simulink library "HybridSimLib"  (Simulink 7.9)
settings: Solver=ode45  SolverMode=SingleTasking  StartTime=0.0  StopTime=10.0  RelTol=1e-3
undefined symbols (not defined in the file or in its folder): DiscIntNeverNeededParam, HybridCtrlParameters, newTarget, targDsp
libraries: simulink x10, xpclib x7
settings Model: Creator=Andreas Schellenberg  LastModifiedBy=Andreas

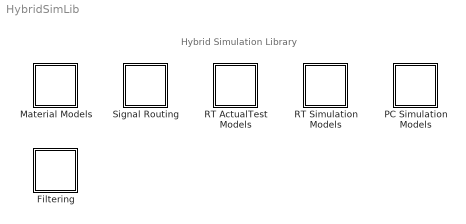
== system HybridSimLib ==
  note: Hybrid Simulation Library
  Filtering : Subsystem
  Material Models : Subsystem
  PC Simulation Models : Subsystem
  RT ActualTest Models : Subsystem
  RT Simulation Models : Subsystem
  Signal Routing : Subsystem

== system HybridSimLib/Filtering ==
  note: Filtering Blocks
  MovingAverage Filter : DiscreteFir  Coefficients=1/numSample*ones(1,numSample)  mask(Moving Average Filter){numSample=5}
      mask prompts: numSample "Number of Samples: numSample"
      mask help:
      | Moving average filter by using discrete FIR filter.
      | Set numSample = 1 for no filtering.
      mask Display: fprintf('MovingAverage\nFilter')
  median filter : S-Function  FunctionName=medianFilter  Parameters=width  EnableBusSupport=off  mask(Moving Median Filter){width=1}
      mask prompts: width "Glitch width (samples)"
      mask Display: fprintf('MovingMedian\nFilter')

== system HybridSimLib/Material Models ==
  note: Material Model Blocks
  continuousD : Subsystem  mask(Continuous Bouc-Wen Model){k=, fy=, alpha=, beta=0.5, gamma=0.5, n=1.0}
      mask prompts: k "Elastic Stiffness: k"; fy "Yield Strength: fy"; alpha "Post-Yield Stiffness Ratio: alpha"; beta "Hysteresis Shape Parameter: beta"; gamma "Hysteresis Shape Parameter: gamma"; n "Smoothness of Transition Parameter: n"
      mask help: Continuous model using displacement inputs to produce force outputs.
      mask Display: disp('Bouc-Wen\nModel')
  continuousDV : Subsystem  mask(Continuous Bouc-Wen Model){k=, fy=, alpha=, beta=0.5, gamma=0.5, n=1.0}
      mask prompts: k "Elastic Stiffness: k"; fy "Yield Strength: fy"; alpha "Post-Yield Stiffness Ratio: alpha"; beta "Hysteresis Shape Parameter: beta"; gamma "Hysteresis Shape Parameter: gamma"; n "Smoothness of Transition Parameter: n"
      mask help: Continuous model using displacement and velocity inputs to produce force outputs.
      mask Display: disp('Bouc-Wen\nModel')
  discreteD : Subsystem  mask(Discrete Bouc-Wen Model){k=, fy=, alpha=, beta=, gamma=0.5, n=0.5, dt=1.0}
      mask prompts: k "Elastic Stiffness: k"; fy "Yield Strength: fy"; alpha "Post-Yield Stiffness Ratio: alpha"; beta "Hysteresis Shape Parameter: beta"; gamma "Hysteresis Shape Parameter: gamma"; n "Smoothness of Transition Parameter: n"; dt "Sample time: dt"
      mask help: Discrete model using displacement inputs to produce force outputs.
      mask Display: disp('Bouc-Wen\nModel')
  discreteDV : Subsystem  mask(Discrete Bouc-Wen Model){k=, fy=, alpha=, beta=0.5, gamma=0.5, n=1.0}
      mask prompts: k "Elastic Stiffness: k"; fy "Yield Strength: fy"; alpha "Post-Yield Stiffness Ratio: alpha"; beta "Hysteresis Shape Parameter: beta"; gamma "Hysteresis Shape Parameter: gamma"; n "Smoothness of Transition Parameter: n"
      mask help: Discrete model using displacement and velocity inputs to produce force outputs.
      mask Display: disp('Bouc-Wen\nModel')

== system HybridSimLib/PC Simulation Models ==
  note: PC Simulation Models
  cmAPI dSpace : Subsystem
  cmAPI xPCTarget STS : Subsystem

== system HybridSimLib/RT ActualTest Models ==
  note: Real Time ActualTest Models
  cmAPI dSpace : Subsystem
  cmAPI xPCTarget STS : Subsystem

== system HybridSimLib/RT Simulation Models ==
  note: Real Time Simulation Models
  cmAPI dSpace : Subsystem
  cmAPI xPCTarget STS : Subsystem

== system HybridSimLib/Signal Routing ==
  note: Signal Routing Blocks
  Offset : Subsystem  mask(Signal Offset){nS=[], nOffset=[], dt=[]}
      mask prompts: nS "Number of Signals: nS"; nOffset "Number of samples to initialize offset: nOffset"; dt "Sample time: dt"
      mask help:
      | Offset signal by average of signal over initial number of samples.
      | Set nOffset = -1 for no signal offset.
      mask Display: fprintf('Signal\nOffset')
  assemble : Subsystem  mask(to Actuators){id=, size=}
      mask prompts: id "Index Vector: id"; size "Vector Size: size"
      mask help: To select to which actuator(s) the signals are going to
      mask Display: disp('Assemble')
  extract : Subsystem  mask(from Actuators){id=, size=}
      mask prompts: id "Index Vector: id"; size "Vector Size: size"
      mask help: To select from which actuator(s) the signals are coming from
      mask Display: disp('Extract')

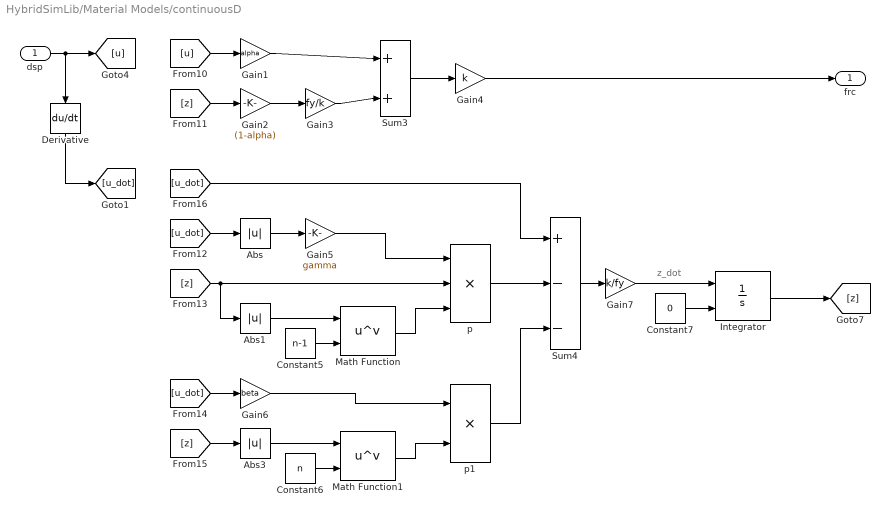
== system HybridSimLib/Material Models/continuousD ==
  note: z_dot
  dsp : Inport
  Abs : Abs  SaturateOnIntegerOverflow=on
  Abs1 : Abs  SaturateOnIntegerOverflow=on
  Abs3 : Abs  SaturateOnIntegerOverflow=on
  Constant5 : Constant  Value=n-1
  Constant6 : Constant  Value=n
  Constant7 : Constant  Value=0
  Derivative : Derivative
  Gain1 : Gain  Gain=alpha  SaturateOnIntegerOverflow=on  OutDataTypeStr=Inherit: Same as input  ParamDataTypeStr=Inherit: Same as input
  Gain2 : Gain  Gain=(1-alpha)  SaturateOnIntegerOverflow=on  OutDataTypeStr=Inherit: Same as input  ParamDataTypeStr=Inherit: Same as input
  Gain3 : Gain  Gain=fy/k  SaturateOnIntegerOverflow=on  OutDataTypeStr=Inherit: Same as input  ParamDataTypeStr=Inherit: Same as input
  Gain4 : Gain  Gain=k  SaturateOnIntegerOverflow=on  OutDataTypeStr=Inherit: Same as input  ParamDataTypeStr=Inherit: Same as input
  Gain5 : Gain  Gain=gamma  SaturateOnIntegerOverflow=on  OutDataTypeStr=Inherit: Same as input  ParamDataTypeStr=Inherit: Same as input
  Gain6 : Gain  Gain=beta  SaturateOnIntegerOverflow=on  OutDataTypeStr=Inherit: Same as input  ParamDataTypeStr=Inherit: Same as input
  Gain7 : Gain  Gain=k/fy  SaturateOnIntegerOverflow=on  OutDataTypeStr=Inherit: Same as input  ParamDataTypeStr=Inherit: Same as input
  Integrator : Integrator  InitialConditionSource=external
  Math Function : Math  Operator=pow  SaturateOnIntegerOverflow=on
  Math Function1 : Math  Operator=pow  SaturateOnIntegerOverflow=on
  Sum3 : Sum  Inputs=+|+  SaturateOnIntegerOverflow=on  InputSameDT=on  OutDataTypeStr=Inherit: Same as first input
  Sum4 : Sum  Inputs=+|-|-  SaturateOnIntegerOverflow=on  InputSameDT=on  OutDataTypeStr=Inherit: Same as first input
  p : Product  Inputs=***  SaturateOnIntegerOverflow=on  InputSameDT=on  OutDataTypeStr=Inherit: Same as first input
  p1 : Product  Inputs=**  SaturateOnIntegerOverflow=on  InputSameDT=on  OutDataTypeStr=Inherit: Same as first input
  frc : Outport
  wires:
  [u] -> Gain1/1
  Gain2/1 -> Gain3/1
  [z] -> Gain2/1
  Gain3/1 -> Sum3/2
  Gain1/1 -> Sum3/1
  Sum3/1 -> Gain4/1
  Gain4/1 -> frc/1
  [u_dot] -> Abs/1
  [z] -> p/2, Abs1/1
  Abs/1 -> Gain5/1
  Abs1/1 -> Math Function/1
  Constant5/1 -> Math Function/2
  Gain5/1 -> p/1
  Math Function/1 -> p/3
  [z] -> Abs3/1
  [u_dot] -> Gain6/1
  Abs3/1 -> Math Function1/1
  Constant6/1 -> Math Function1/2
  Gain6/1 -> p1/1
  Math Function1/1 -> p1/2
  p/1 -> Sum4/2
  p1/1 -> Sum4/3
  [u_dot] -> Sum4/1
  Constant7/1 -> Integrator/2
  Sum4/1 -> Gain7/1
  Integrator/1 -> [z]
  dsp/1 -> [u], Derivative/1
  Derivative/1 -> [u_dot]
  Gain7/1 -> Integrator/1

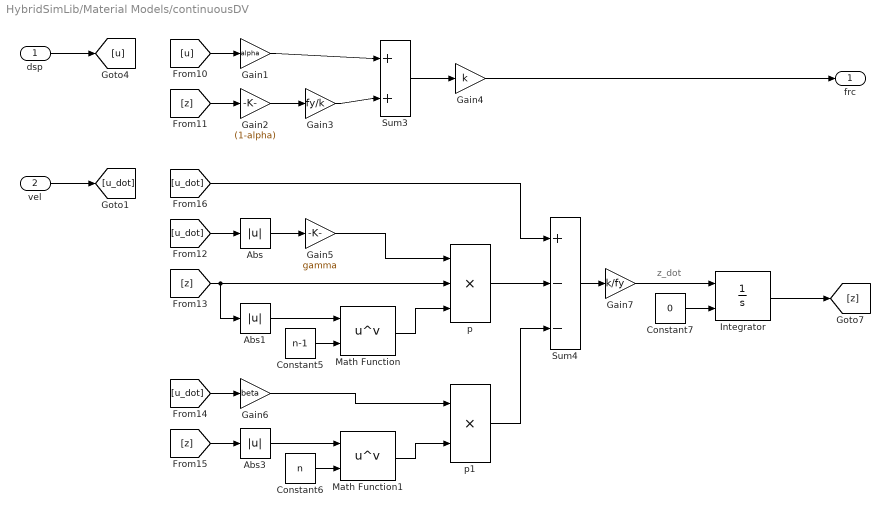
== system HybridSimLib/Material Models/continuousDV ==
  note: z_dot
  dsp : Inport
  vel : Inport  Port=2
  Abs : Abs  SaturateOnIntegerOverflow=on
  Abs1 : Abs  SaturateOnIntegerOverflow=on
  Abs3 : Abs  SaturateOnIntegerOverflow=on
  Constant5 : Constant  Value=n-1
  Constant6 : Constant  Value=n
  Constant7 : Constant  Value=0
  Gain1 : Gain  Gain=alpha  SaturateOnIntegerOverflow=on  OutDataTypeStr=Inherit: Same as input  ParamDataTypeStr=Inherit: Same as input
  Gain2 : Gain  Gain=(1-alpha)  SaturateOnIntegerOverflow=on  OutDataTypeStr=Inherit: Same as input  ParamDataTypeStr=Inherit: Same as input
  Gain3 : Gain  Gain=fy/k  SaturateOnIntegerOverflow=on  OutDataTypeStr=Inherit: Same as input  ParamDataTypeStr=Inherit: Same as input
  Gain4 : Gain  Gain=k  SaturateOnIntegerOverflow=on  OutDataTypeStr=Inherit: Same as input  ParamDataTypeStr=Inherit: Same as input
  Gain5 : Gain  Gain=gamma  SaturateOnIntegerOverflow=on  OutDataTypeStr=Inherit: Same as input  ParamDataTypeStr=Inherit: Same as input
  Gain6 : Gain  Gain=beta  SaturateOnIntegerOverflow=on  OutDataTypeStr=Inherit: Same as input  ParamDataTypeStr=Inherit: Same as input
  Gain7 : Gain  Gain=k/fy  SaturateOnIntegerOverflow=on  OutDataTypeStr=Inherit: Same as input  ParamDataTypeStr=Inherit: Same as input
  Integrator : Integrator  InitialConditionSource=external
  Math Function : Math  Operator=pow  SaturateOnIntegerOverflow=on
  Math Function1 : Math  Operator=pow  SaturateOnIntegerOverflow=on
  Sum3 : Sum  Inputs=+|+  SaturateOnIntegerOverflow=on  InputSameDT=on  OutDataTypeStr=Inherit: Same as first input
  Sum4 : Sum  Inputs=+|-|-  SaturateOnIntegerOverflow=on  InputSameDT=on  OutDataTypeStr=Inherit: Same as first input
  p : Product  Inputs=***  SaturateOnIntegerOverflow=on  InputSameDT=on  OutDataTypeStr=Inherit: Same as first input
  p1 : Product  Inputs=**  SaturateOnIntegerOverflow=on  InputSameDT=on  OutDataTypeStr=Inherit: Same as first input
  frc : Outport
  wires:
  Gain7/1 -> Integrator/1
  dsp/1 -> [u]
  Integrator/1 -> [z]
  Sum4/1 -> Gain7/1
  Constant7/1 -> Integrator/2
  [u_dot] -> Sum4/1
  p1/1 -> Sum4/3
  p/1 -> Sum4/2
  Math Function1/1 -> p1/2
  Gain6/1 -> p1/1
  Constant6/1 -> Math Function1/2
  Abs3/1 -> Math Function1/1
  [u_dot] -> Gain6/1
  [z] -> Abs3/1
  Math Function/1 -> p/3
  Gain5/1 -> p/1
  Constant5/1 -> Math Function/2
  Abs1/1 -> Math Function/1
  Abs/1 -> Gain5/1
  [z] -> Abs1/1, p/2
  [u_dot] -> Abs/1
  Gain4/1 -> frc/1
  Sum3/1 -> Gain4/1
  Gain1/1 -> Sum3/1
  Gain3/1 -> Sum3/2
  [z] -> Gain2/1
  Gain2/1 -> Gain3/1
  [u] -> Gain1/1
  vel/1 -> [u_dot]

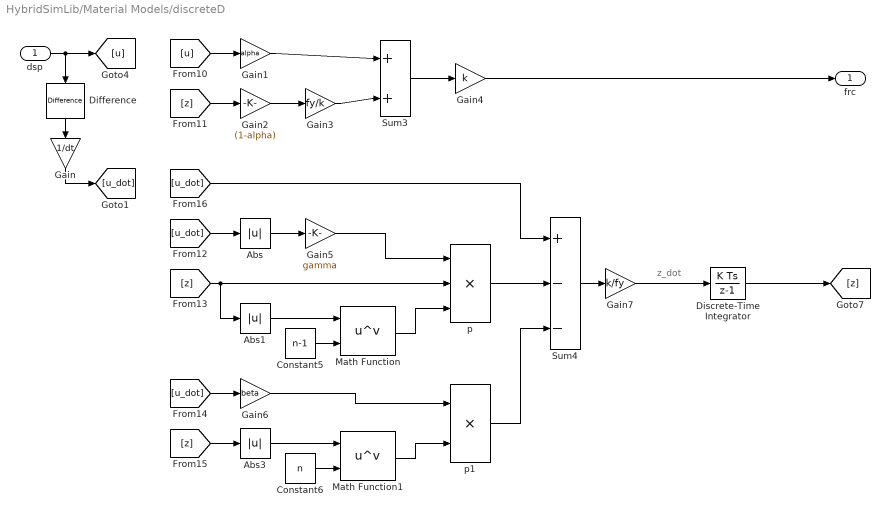
== system HybridSimLib/Material Models/discreteD ==
  note: z_dot
  dsp : Inport
  Abs : Abs  SaturateOnIntegerOverflow=on
  Abs1 : Abs  SaturateOnIntegerOverflow=on
  Abs3 : Abs  SaturateOnIntegerOverflow=on
  Constant5 : Constant  Value=n-1
  Constant6 : Constant  Value=n
  Difference : simulink/Discrete/Difference  ICPrevInput=0.0  InputProcessing=Inherited  OutMin=[]  OutMax=[]  OutDataType=sfix(16)  OutScaling=2^-10  DoSatur=off
  Discrete-Time Integrator : DiscreteIntegrator  SampleTime=-1  ICPrevOutput=DiscIntNeverNeededParam  ICPrevScaledInput=DiscIntNeverNeededParam
  Gain : Gain  Gain=1/dt
  Gain1 : Gain  Gain=alpha  SaturateOnIntegerOverflow=on  OutDataTypeStr=Inherit: Same as input  ParamDataTypeStr=Inherit: Same as input
  Gain2 : Gain  Gain=(1-alpha)  SaturateOnIntegerOverflow=on  OutDataTypeStr=Inherit: Same as input  ParamDataTypeStr=Inherit: Same as input
  Gain3 : Gain  Gain=fy/k  SaturateOnIntegerOverflow=on  OutDataTypeStr=Inherit: Same as input  ParamDataTypeStr=Inherit: Same as input
  Gain4 : Gain  Gain=k  SaturateOnIntegerOverflow=on  OutDataTypeStr=Inherit: Same as input  ParamDataTypeStr=Inherit: Same as input
  Gain5 : Gain  Gain=gamma  SaturateOnIntegerOverflow=on  OutDataTypeStr=Inherit: Same as input  ParamDataTypeStr=Inherit: Same as input
  Gain6 : Gain  Gain=beta  SaturateOnIntegerOverflow=on  OutDataTypeStr=Inherit: Same as input  ParamDataTypeStr=Inherit: Same as input
  Gain7 : Gain  Gain=k/fy  SaturateOnIntegerOverflow=on  OutDataTypeStr=Inherit: Same as input  ParamDataTypeStr=Inherit: Same as input
  Math Function : Math  Operator=pow  SaturateOnIntegerOverflow=on
  Math Function1 : Math  Operator=pow  SaturateOnIntegerOverflow=on
  Sum3 : Sum  Inputs=+|+  SaturateOnIntegerOverflow=on  InputSameDT=on  OutDataTypeStr=Inherit: Same as first input
  Sum4 : Sum  Inputs=+|-|-  SaturateOnIntegerOverflow=on  InputSameDT=on  OutDataTypeStr=Inherit: Same as first input
  p : Product  Inputs=***  SaturateOnIntegerOverflow=on  InputSameDT=on  OutDataTypeStr=Inherit: Same as first input
  p1 : Product  Inputs=**  SaturateOnIntegerOverflow=on  InputSameDT=on  OutDataTypeStr=Inherit: Same as first input
  frc : Outport
  wires:
  [u] -> Gain1/1
  Gain2/1 -> Gain3/1
  [z] -> Gain2/1
  Gain3/1 -> Sum3/2
  Gain1/1 -> Sum3/1
  Sum3/1 -> Gain4/1
  Gain4/1 -> frc/1
  [u_dot] -> Abs/1
  [z] -> p/2, Abs1/1
  Abs/1 -> Gain5/1
  Abs1/1 -> Math Function/1
  Constant5/1 -> Math Function/2
  Gain5/1 -> p/1
  Math Function/1 -> p/3
  [z] -> Abs3/1
  [u_dot] -> Gain6/1
  Abs3/1 -> Math Function1/1
  Constant6/1 -> Math Function1/2
  Gain6/1 -> p1/1
  Math Function1/1 -> p1/2
  p/1 -> Sum4/2
  p1/1 -> Sum4/3
  [u_dot] -> Sum4/1
  Sum4/1 -> Gain7/1
  Discrete-Time Integrator/1 -> [z]
  dsp/1 -> [u], Difference/1
  Gain7/1 -> Discrete-Time Integrator/1
  Difference/1 -> Gain/1
  Gain/1 -> [u_dot]

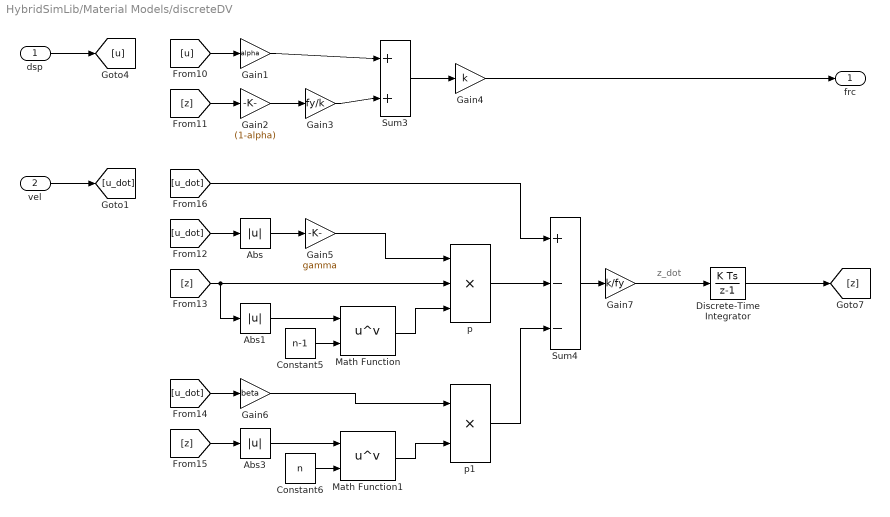
== system HybridSimLib/Material Models/discreteDV ==
  note: z_dot
  dsp : Inport
  vel : Inport  Port=2
  Abs : Abs  SaturateOnIntegerOverflow=on
  Abs1 : Abs  SaturateOnIntegerOverflow=on
  Abs3 : Abs  SaturateOnIntegerOverflow=on
  Constant5 : Constant  Value=n-1
  Constant6 : Constant  Value=n
  Discrete-Time Integrator : DiscreteIntegrator  SampleTime=-1  ICPrevOutput=DiscIntNeverNeededParam  ICPrevScaledInput=DiscIntNeverNeededParam
  Gain1 : Gain  Gain=alpha  SaturateOnIntegerOverflow=on  OutDataTypeStr=Inherit: Same as input  ParamDataTypeStr=Inherit: Same as input
  Gain2 : Gain  Gain=(1-alpha)  SaturateOnIntegerOverflow=on  OutDataTypeStr=Inherit: Same as input  ParamDataTypeStr=Inherit: Same as input
  Gain3 : Gain  Gain=fy/k  SaturateOnIntegerOverflow=on  OutDataTypeStr=Inherit: Same as input  ParamDataTypeStr=Inherit: Same as input
  Gain4 : Gain  Gain=k  SaturateOnIntegerOverflow=on  OutDataTypeStr=Inherit: Same as input  ParamDataTypeStr=Inherit: Same as input
  Gain5 : Gain  Gain=gamma  SaturateOnIntegerOverflow=on  OutDataTypeStr=Inherit: Same as input  ParamDataTypeStr=Inherit: Same as input
  Gain6 : Gain  Gain=beta  SaturateOnIntegerOverflow=on  OutDataTypeStr=Inherit: Same as input  ParamDataTypeStr=Inherit: Same as input
  Gain7 : Gain  Gain=k/fy  SaturateOnIntegerOverflow=on  OutDataTypeStr=Inherit: Same as input  ParamDataTypeStr=Inherit: Same as input
  Math Function : Math  Operator=pow  SaturateOnIntegerOverflow=on
  Math Function1 : Math  Operator=pow  SaturateOnIntegerOverflow=on
  Sum3 : Sum  Inputs=+|+  SaturateOnIntegerOverflow=on  InputSameDT=on  OutDataTypeStr=Inherit: Same as first input
  Sum4 : Sum  Inputs=+|-|-  SaturateOnIntegerOverflow=on  InputSameDT=on  OutDataTypeStr=Inherit: Same as first input
  p : Product  Inputs=***  SaturateOnIntegerOverflow=on  InputSameDT=on  OutDataTypeStr=Inherit: Same as first input
  p1 : Product  Inputs=**  SaturateOnIntegerOverflow=on  InputSameDT=on  OutDataTypeStr=Inherit: Same as first input
  frc : Outport
  wires:
  vel/1 -> [u_dot]
  [u] -> Gain1/1
  Gain2/1 -> Gain3/1
  [z] -> Gain2/1
  Gain3/1 -> Sum3/2
  Gain1/1 -> Sum3/1
  Sum3/1 -> Gain4/1
  Gain4/1 -> frc/1
  [u_dot] -> Abs/1
  [z] -> p/2, Abs1/1
  Abs/1 -> Gain5/1
  Abs1/1 -> Math Function/1
  Constant5/1 -> Math Function/2
  Gain5/1 -> p/1
  Math Function/1 -> p/3
  [z] -> Abs3/1
  [u_dot] -> Gain6/1
  Abs3/1 -> Math Function1/1
  Constant6/1 -> Math Function1/2
  Gain6/1 -> p1/1
  Math Function1/1 -> p1/2
  p/1 -> Sum4/2
  p1/1 -> Sum4/3
  [u_dot] -> Sum4/1
  Sum4/1 -> Gain7/1
  Discrete-Time Integrator/1 -> [z]
  dsp/1 -> [u]
  Gain7/1 -> Discrete-Time Integrator/1

== system HybridSimLib/PC Simulation Models/cmAPI dSpace ==
  note: cmAPI-dSpace Blocks

== system HybridSimLib/PC Simulation Models/cmAPI xPCTarget STS ==
  note: cmAPI-xPCTarget-STS Blocks

== system HybridSimLib/RT ActualTest Models/cmAPI dSpace ==
  note: cmAPI-dSpace Blocks
  dSpace HC : Subsystem  mask(Hybrid Controller: D3/D3){nAct=1, dtInt=HybridCtrlParameters.dtInt, dtSim=HybridCtrlParameters.dtSim, dtCon=HybridCtrlParameters.dtCon, N=HybridCtrlParameters.N, iDelay=HybridCtrlParameters.iDelay, dspLim=HybridCtrlParameters.dspLim, velLim=HybridCtrlParameters.velLim}
      mask prompts: nAct "Number of Actuators: nAct"; dtInt "Integration time step: dtInt"; dtSim "Simulation time step: dtSim"; dtCon "Controller time step: dtCon"; N "Maximum number of substeps: N"; iDelay "Number of delay steps: iDelay"; dspLim "Displacement limit: dspLim"; velLim "Velocity limit: velLim"
      mask help: Hybrid Controller using C0-continuous cubic Lagrange interpolation for prediction and correction
      mask Display: disp('dSpace\nHybrid Controller\n(D3/D3)')

== system HybridSimLib/RT ActualTest Models/cmAPI xPCTarget STS ==
  note: cmAPI-xPCTarget-STS Blocks
  xPC HC : Subsystem  mask(Hybrid Controller: D3/D3){nAct=1, dtInt=HybridCtrlParameters.dtInt, dtSim=HybridCtrlParameters.dtSim, dtCon=HybridCtrlParameters.dtCon, N=HybridCtrlParameters.N, iDelay=HybridCtrlParameters.iDelay}
      mask prompts: nAct "Number of Actuators: nAct"; dtInt "Integration time step: dtInt"; dtSim "Simulation time step: dtSim"; dtCon "Controller time step: dtCon"; N "Maximum number of substeps: N"; iDelay "Number of delay steps: iDelay"
      mask help: Hybrid Controller using C0-continuous cubic Lagrange interpolation for prediction and correction
      mask Display: disp('xPC Target\nHybrid Controller\n(D3/D3)')

== system HybridSimLib/RT Simulation Models/cmAPI dSpace ==
  note: cmAPI-dSpace Blocks

== system HybridSimLib/RT Simulation Models/cmAPI xPCTarget STS ==
  note: cmAPI-xPCTarget-STS Blocks

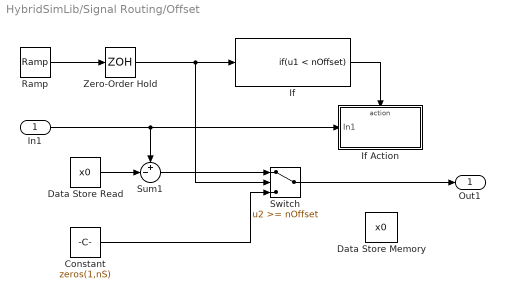
== system HybridSimLib/Signal Routing/Offset ==
  In1 : Inport
  Constant : Constant  Value=zeros(1,nS)
  Data Store Memory : DataStoreMemory  DataStoreName=x0  InitialValue=zeros(1,nS)  OutDataTypeStr=double
  Data Store Read : DataStoreRead  DataStoreName=x0  SampleTime=dt
  If : If  IfExpression=u1 < nOffset  ShowElse=off
  If Action : Subsystem  TreatAsAtomicUnit=on
  Ramp : simulink/Sources/Ramp  slope=1/dt  start=0  X0=0
  Sum1 : Sum  Inputs=+-|  SaturateOnIntegerOverflow=on  InputSameDT=on  OutDataTypeStr=Inherit: Same as first input
  Switch : Switch  Threshold=nOffset  SaturateOnIntegerOverflow=on  InputSameDT=on
  Zero-Order Hold : ZeroOrderHold  SampleTime=dt
  Out1 : Outport
  wires:
  Ramp/1 -> Zero-Order Hold/1
  If/1 -> If Action/Action
  Zero-Order Hold/1 -> If/1, Switch/2
  Constant/1 -> Switch/3
  In1/1 -> Sum1/1, If Action/1(In1)
  Data Store Read/1 -> Sum1/2
  Sum1/1 -> Switch/1
  Switch/1 -> Out1/1

== system HybridSimLib/Signal Routing/assemble ==
  In1 : Inport
  Assignment : Assignment  OutputInitialize=Specify size for each dimension in table  IndexOptions=Index vector (port)  Indices=1  OutputSizes=size
  Constant : Constant  Value=id
  Out1 : Outport
  wires:
  In1/1 -> Assignment/1
  Assignment/1 -> Out1/1
  Constant/1 -> Assignment/2

== system HybridSimLib/Signal Routing/extract ==
  In1 : Inport
  Selector : Selector  InputPortWidth=size  IndexOptions=Index vector (dialog)  Indices=id  OutputSizes=1
  Out1 : Outport
  wires:
  In1/1 -> Selector/1
  Selector/1 -> Out1/1

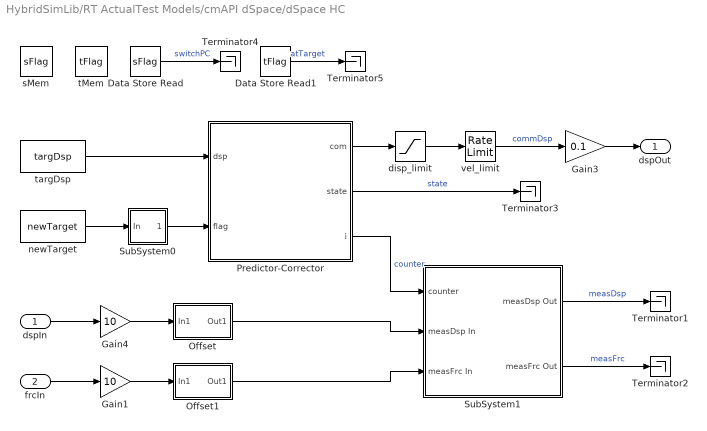
== system HybridSimLib/RT ActualTest Models/cmAPI dSpace/dSpace HC ==
  dspIn : Inport
  frcIn : Inport  Port=2
  Data Store Read : DataStoreRead  DataStoreName=sFlag  SampleTime=dtCon
  Data Store Read1 : DataStoreRead  DataStoreName=tFlag  SampleTime=dtCon
  Gain1 : Gain  Gain=10  SaturateOnIntegerOverflow=on  OutDataTypeStr=Inherit: Same as input  ParamDataTypeStr=Inherit: Same as input
  Gain3 : Gain  Gain=0.1  SaturateOnIntegerOverflow=on  OutDataTypeStr=Inherit: Same as input  ParamDataTypeStr=Inherit: Same as input
  Gain4 : Gain  Gain=10  SaturateOnIntegerOverflow=on  OutDataTypeStr=Inherit: Same as input  ParamDataTypeStr=Inherit: Same as input
  Offset : Subsystem  mask(Signal Offset){nS=nAct, nOffset=1024, dt=dtCon}
      mask prompts: nS "Number of Signals: nS"; nOffset "Number of samples to initialize offset: nOffset"; dt "Sample time: dt"
      mask help: Offset signal by average of signal over initial number of samples
      mask Display: fprintf('Signal\nOffset')
  Offset1 : Subsystem  mask(Signal Offset){nS=nAct, nOffset=1024, dt=dtCon}
      mask prompts: nS "Number of Signals: nS"; nOffset "Number of samples to initialize offset: nOffset"; dt "Sample time: dt"
      mask help: Offset signal by average of signal over initial number of samples
      mask Display: fprintf('Signal\nOffset')
  Predictor-Corrector : Stateflow chart  TreatAsAtomicUnit=on
  SubSystem0 : Subsystem
  SubSystem1 : Subsystem
  Terminator{1..5} (5 alike) : Terminator
  disp_limit : Saturate  UpperLimit=dspLim  LowerLimit=-dspLim
  newTarget : Constant  Value=newTarget  OutDataTypeStr=uint32  SampleTime=dtCon
  sMem : DataStoreMemory  DataStoreName=sFlag  OutDataTypeStr=uint32
  tMem : DataStoreMemory  DataStoreName=tFlag  OutDataTypeStr=uint32
  targDsp : Constant  Value=targDsp  SampleTime=dtCon
  vel_limit : RateLimiter  RisingSlewLimit=velLim  FallingSlewLimit=-velLim
  dspOut : Outport
  wires:
  Data Store Read1/1 -> Terminator5/1  "atTarget"
  Data Store Read/1 -> Terminator4/1  "switchPC"
  Gain1/1 -> Offset1/1(In1)
  Gain4/1 -> Offset/1(In1)
  Gain3/1 -> dspOut/1
  Predictor-Corrector/1(com) -> disp_limit/1
  vel_limit/1 -> Gain3/1  "commDsp"
  disp_limit/1 -> vel_limit/1
  Offset1/1(Out1) -> SubSystem1/3(measFrc In)
  targDsp/1 -> Predictor-Corrector/1(dsp)
  newTarget/1 -> SubSystem0/1(In)
  SubSystem0/1(Out) -> Predictor-Corrector/2(flag)
  Offset/1(Out1) -> SubSystem1/2(measDsp In)
  Predictor-Corrector/2(state) -> Terminator3/1  "state"
  Predictor-Corrector/3(i) -> SubSystem1/1(counter)  "counter"
  SubSystem1/1(measDsp Out) -> Terminator1/1  "measDsp"
  SubSystem1/2(measFrc Out) -> Terminator2/1  "measFrc"
  dspIn/1 -> Gain4/1
  frcIn/1 -> Gain1/1

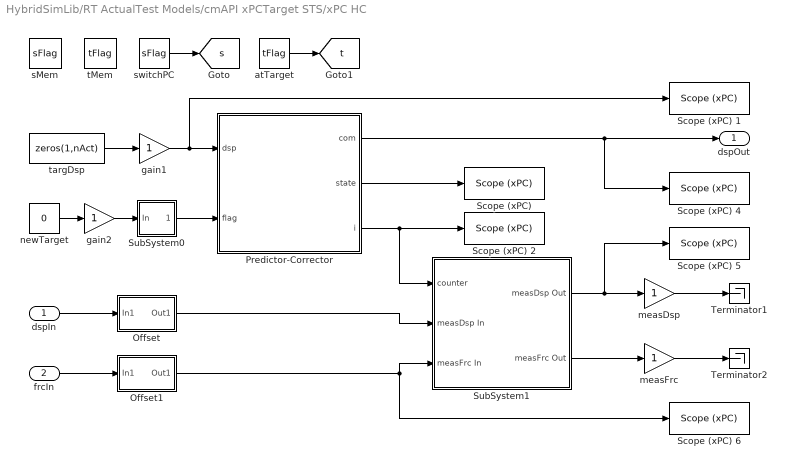
== system HybridSimLib/RT ActualTest Models/cmAPI xPCTarget STS/xPC HC ==
  dspIn : Inport
  frcIn : Inport  Port=2
  Offset : Subsystem  mask(Signal Offset){nS=nAct, nOffset=1024, dt=dtCon}
      mask prompts: nS "Number of Signals: nS"; nOffset "Number of samples to initialize offset: nOffset"; dt "Sample time: dt"
      mask help: Offset signal by average of signal over initial number of samples
      mask Display: fprintf('Signal\nOffset')
  Offset1 : Subsystem  mask(Signal Offset){nS=nAct, nOffset=1024, dt=dtCon}
      mask prompts: nS "Number of Signals: nS"; nOffset "Number of samples to initialize offset: nOffset"; dt "Sample time: dt"
      mask help: Offset signal by average of signal over initial number of samples
      mask Display: fprintf('Signal\nOffset')
  Predictor-Corrector : Stateflow chart  TreatAsAtomicUnit=on
  "Scope (xPC) " : xpclib/Misc./Scope (xPC)   scopeno=4  scopetype=File  autostart=on  viewmode=Graphical redraw  formatstr='%15.6f'  grid=on  ylimits=[0,3]  nosamples=4096  noprepostsamples=0  interleave=1  triggermode=FreeRun  triggersignal=1  triggerlevel=0.0  triggerslope=Either  triggerscope=1  triggersample=0  filename=state.dat  mode=Lazy  writesize=512  autorestart=on  dynamicfilemode=off  maxwritefilesize=512*1024^2
  Scope (xPC) 1 : xpclib/Misc./Scope (xPC)   scopeno=1  scopetype=File  autostart=on  viewmode=Numerical  formatstr='%15.6f'  grid=on  ylimits=[-4,4]  nosamples=4096  noprepostsamples=0  interleave=1  triggermode=FreeRun  triggersignal=1  triggerlevel=0.0  triggerslope=Either  triggerscope=1  triggersample=0  filename=targDsp.dat  mode=Lazy  writesize=512  autorestart=on  dynamicfilemode=off  maxwritefilesize=512*1024^2
  Scope (xPC) 2 : xpclib/Misc./Scope (xPC)   scopeno=5  scopetype=File  autostart=on  viewmode=Numerical  formatstr='%15.6f'  grid=on  ylimits=[0,3]  nosamples=4096  noprepostsamples=0  interleave=1  triggermode=FreeRun  triggersignal=1  triggerlevel=0.0  triggerslope=Either  triggerscope=1  triggersample=0  filename=count.dat  mode=Lazy  writesize=512  autorestart=on  dynamicfilemode=off  maxwritefilesize=512*1024^2
  Scope (xPC) 4 : xpclib/Misc./Scope (xPC)   scopeno=2  scopetype=File  autostart=on  viewmode=Numerical  formatstr='%15.6f'  grid=on  ylimits=[-4,4]  nosamples=4096  noprepostsamples=0  interleave=1  triggermode=FreeRun  triggersignal=1  triggerlevel=0.0  triggerslope=Either  triggerscope=1  triggersample=0  filename=commDsp.dat  mode=Lazy  writesize=512  autorestart=on  dynamicfilemode=off  maxwritefilesize=512*1024^2
  Scope (xPC) 5 : xpclib/Misc./Scope (xPC)   scopeno=3  scopetype=File  autostart=on  viewmode=Numerical  formatstr='%15.6f'  grid=on  ylimits=[-4,4]  nosamples=4096  noprepostsamples=0  interleave=1  triggermode=FreeRun  triggersignal=1  triggerlevel=0.0  triggerslope=Either  triggerscope=1  triggersample=0  filename=measDsp.dat  mode=Lazy  writesize=512  autorestart=on  dynamicfilemode=off  maxwritefilesize=512*1024^2
  Scope (xPC) 6 : xpclib/Misc./Scope (xPC)   scopeno=6  scopetype=File  autostart=on  viewmode=Numerical  formatstr='%15.6f'  grid=on  ylimits=[0,3]  nosamples=4096  noprepostsamples=0  interleave=1  triggermode=FreeRun  triggersignal=1  triggerlevel=0.0  triggerslope=Either  triggerscope=1  triggersample=0  filename=measFrc.dat  mode=Lazy  writesize=512  autorestart=on  dynamicfilemode=off  maxwritefilesize=512*1024^2
  SubSystem0 : Subsystem
  SubSystem1 : Subsystem
  Terminator1 : Terminator
  Terminator2 : Terminator
  atTarget : DataStoreRead  DataStoreName=tFlag  SampleTime=dtCon
  gain1 : Gain
  gain2 : Gain
  measDsp : Gain
  measFrc : Gain
  newTarget : Constant  Value=0  SampleTime=dtCon
  sMem : DataStoreMemory  DataStoreName=sFlag  OutDataTypeStr=double
  switchPC : DataStoreRead  DataStoreName=sFlag  SampleTime=dtCon
  tMem : DataStoreMemory  DataStoreName=tFlag  OutDataTypeStr=double
  targDsp : Constant  Value=zeros(1,nAct)  SampleTime=dtCon
  dspOut : Outport
  tag scope: s=global, t=global
  wires:
  Offset1/1(Out1) -> SubSystem1/3(measFrc In), Scope (xPC) 6/1
  gain1/1 -> Scope (xPC) 1/1, Predictor-Corrector/1(dsp)
  targDsp/1 -> gain1/1
  atTarget/1 -> [t]
  switchPC/1 -> [s]
  gain2/1 -> SubSystem0/1(In)
  newTarget/1 -> gain2/1
  SubSystem0/1(Out) -> Predictor-Corrector/2(flag)
  Offset/1(Out1) -> SubSystem1/2(measDsp In)
  Predictor-Corrector/1(com) -> Scope (xPC) 4/1, dspOut/1
  Predictor-Corrector/2(state) -> "Scope (xPC) "/1
  Predictor-Corrector/3(i) -> Scope (xPC) 2/1, SubSystem1/1(counter)
  SubSystem1/1(measDsp Out) -> Scope (xPC) 5/1, measDsp/1
  SubSystem1/2(measFrc Out) -> measFrc/1
  dspIn/1 -> Offset/1(In1)
  measDsp/1 -> Terminator1/1
  measFrc/1 -> Terminator2/1
  frcIn/1 -> Offset1/1(In1)

== system HybridSimLib/Signal Routing/Offset/If Action ==
  In1 : Inport
  Action Port : ActionPort  PropagateVarSize=During execution
  Data Store Read : DataStoreRead  DataStoreName=x0  SampleTime=dt
  Data Store Write : DataStoreWrite  DataStoreName=x0
  Gain : Gain  Gain=1/nOffset  SaturateOnIntegerOverflow=on  OutDataTypeStr=Inherit: Same as input  ParamDataTypeStr=Inherit: Same as input
  Sum : Sum  Inputs=|++  SaturateOnIntegerOverflow=on  InputSameDT=on  OutDataTypeStr=Inherit: Same as first input
  wires:
  In1/1 -> Gain/1
  Gain/1 -> Sum/1
  Sum/1 -> Data Store Write/1
  Data Store Read/1 -> Sum/2

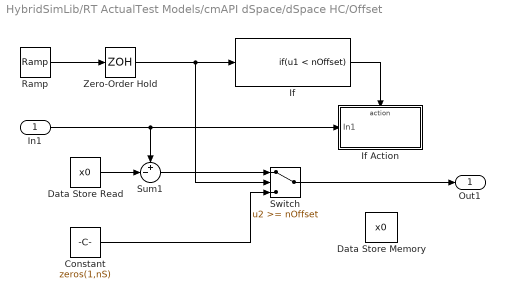
== system HybridSimLib/RT ActualTest Models/cmAPI dSpace/dSpace HC/Offset ==
  In1 : Inport
  Constant : Constant  Value=zeros(1,nS)
  Data Store Memory : DataStoreMemory  DataStoreName=x0  InitialValue=zeros(1,nS)  OutDataTypeStr=double
  Data Store Read : DataStoreRead  DataStoreName=x0  SampleTime=dt
  If : If  IfExpression=u1 < nOffset  ShowElse=off
  If Action : Subsystem  TreatAsAtomicUnit=on
  Ramp : simulink/Sources/Ramp  slope=1/dt  start=0  X0=0
  Sum1 : Sum  Inputs=+-|  SaturateOnIntegerOverflow=on  InputSameDT=on  OutDataTypeStr=Inherit: Same as first input
  Switch : Switch  Threshold=nOffset  SaturateOnIntegerOverflow=on  InputSameDT=on
  Zero-Order Hold : ZeroOrderHold  SampleTime=dt
  Out1 : Outport
  wires:
  Ramp/1 -> Zero-Order Hold/1
  If/1 -> If Action/Action
  Zero-Order Hold/1 -> If/1, Switch/2
  Constant/1 -> Switch/3
  In1/1 -> Sum1/1, If Action/1(In1)
  Data Store Read/1 -> Sum1/2
  Sum1/1 -> Switch/1
  Switch/1 -> Out1/1

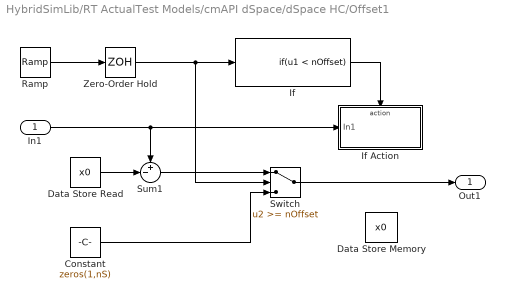
== system HybridSimLib/RT ActualTest Models/cmAPI dSpace/dSpace HC/Offset1 ==
  In1 : Inport
  Constant : Constant  Value=zeros(1,nS)
  Data Store Memory : DataStoreMemory  DataStoreName=x0  InitialValue=zeros(1,nS)  OutDataTypeStr=double
  Data Store Read : DataStoreRead  DataStoreName=x0  SampleTime=dt
  If : If  IfExpression=u1 < nOffset  ShowElse=off
  If Action : Subsystem  TreatAsAtomicUnit=on
  Ramp : simulink/Sources/Ramp  slope=1/dt  start=0  X0=0
  Sum1 : Sum  Inputs=+-|  SaturateOnIntegerOverflow=on  InputSameDT=on  OutDataTypeStr=Inherit: Same as first input
  Switch : Switch  Threshold=nOffset  SaturateOnIntegerOverflow=on  InputSameDT=on
  Zero-Order Hold : ZeroOrderHold  SampleTime=dt
  Out1 : Outport
  wires:
  Ramp/1 -> Zero-Order Hold/1
  If/1 -> If Action/Action
  Zero-Order Hold/1 -> If/1, Switch/2
  Constant/1 -> Switch/3
  In1/1 -> Sum1/1, If Action/1(In1)
  Data Store Read/1 -> Sum1/2
  Sum1/1 -> Switch/1
  Switch/1 -> Out1/1

== system HybridSimLib/RT ActualTest Models/cmAPI dSpace/dSpace HC/SubSystem0 ==
  In : Inport
  Detect Fall Nonpositive : simulink/Logic and Bit Operations/Detect Fall Nonpositive  vinit=0  InputProcessing=Inherited  OutDataTypeStr=uint8
  Detect Rise Positive : simulink/Logic and Bit Operations/Detect Rise Positive  vinit=0  InputProcessing=Inherited  OutDataTypeStr=uint8
  If Action Subsystem0 : Subsystem  TreatAsAtomicUnit=on
  If Action Subsystem1 : Subsystem  TreatAsAtomicUnit=on
  If0 : If  IfExpression=u1 == 1  ShowElse=off
  If1 : If  IfExpression=u1 == 1  ShowElse=off
  typeConv : DataTypeConversion  OutDataTypeStr=uint32  SaturateOnIntegerOverflow=on  RndMeth=Zero
  Out : Outport
  wires:
  typeConv/1 -> Out/1
  If0/1 -> If Action Subsystem0/Action
  If1/1 -> If Action Subsystem1/Action
  Detect Fall Nonpositive/1 -> If1/1
  Detect Rise Positive/1 -> typeConv/1, If0/1
  In/1 -> Detect Fall Nonpositive/1, Detect Rise Positive/1  "newTarget"

== system HybridSimLib/RT ActualTest Models/cmAPI dSpace/dSpace HC/SubSystem1 ==
  counter : Inport
  measDsp In : Inport  Port=2
  measFrc In : Inport  Port=3
  Hit  Crossing : HitCross  HitCrossingOffset=iDelay
  SubSystem : Subsystem  TreatAsAtomicUnit=on
  measDsp Out : Outport
  measFrc Out : Outport  Port=2
  wires:
  Hit  Crossing/1 -> SubSystem/Trigger
  counter/1 -> Hit  Crossing/1
  measDsp In/1 -> SubSystem/1(measDsp In)
  SubSystem/1(measDsp Out) -> measDsp Out/1
  measFrc In/1 -> SubSystem/2(measFrc In)
  SubSystem/2(measFrc Out) -> measFrc Out/1

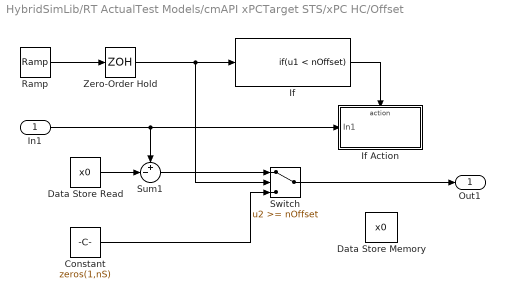
== system HybridSimLib/RT ActualTest Models/cmAPI xPCTarget STS/xPC HC/Offset ==
  In1 : Inport
  Constant : Constant  Value=zeros(1,nS)
  Data Store Memory : DataStoreMemory  DataStoreName=x0  InitialValue=zeros(1,nS)  OutDataTypeStr=double
  Data Store Read : DataStoreRead  DataStoreName=x0  SampleTime=dt
  If : If  IfExpression=u1 < nOffset  ShowElse=off
  If Action : Subsystem  TreatAsAtomicUnit=on
  Ramp : simulink/Sources/Ramp  slope=1/dt  start=0  X0=0
  Sum1 : Sum  Inputs=+-|  SaturateOnIntegerOverflow=on  InputSameDT=on  OutDataTypeStr=Inherit: Same as first input
  Switch : Switch  Threshold=nOffset  SaturateOnIntegerOverflow=on  InputSameDT=on
  Zero-Order Hold : ZeroOrderHold  SampleTime=dt
  Out1 : Outport
  wires:
  Ramp/1 -> Zero-Order Hold/1
  If/1 -> If Action/Action
  Zero-Order Hold/1 -> If/1, Switch/2
  Constant/1 -> Switch/3
  In1/1 -> Sum1/1, If Action/1(In1)
  Data Store Read/1 -> Sum1/2
  Sum1/1 -> Switch/1
  Switch/1 -> Out1/1

== system HybridSimLib/RT ActualTest Models/cmAPI xPCTarget STS/xPC HC/Offset1 ==
  In1 : Inport
  Constant : Constant  Value=zeros(1,nS)
  Data Store Memory : DataStoreMemory  DataStoreName=x0  InitialValue=zeros(1,nS)  OutDataTypeStr=double
  Data Store Read : DataStoreRead  DataStoreName=x0  SampleTime=dt
  If : If  IfExpression=u1 < nOffset  ShowElse=off
  If Action : Subsystem  TreatAsAtomicUnit=on
  Ramp : simulink/Sources/Ramp  slope=1/dt  start=0  X0=0
  Sum1 : Sum  Inputs=+-|  SaturateOnIntegerOverflow=on  InputSameDT=on  OutDataTypeStr=Inherit: Same as first input
  Switch : Switch  Threshold=nOffset  SaturateOnIntegerOverflow=on  InputSameDT=on
  Zero-Order Hold : ZeroOrderHold  SampleTime=dt
  Out1 : Outport
  wires:
  Ramp/1 -> Zero-Order Hold/1
  If/1 -> If Action/Action
  Zero-Order Hold/1 -> If/1, Switch/2
  Constant/1 -> Switch/3
  In1/1 -> Sum1/1, If Action/1(In1)
  Data Store Read/1 -> Sum1/2
  Sum1/1 -> Switch/1
  Switch/1 -> Out1/1

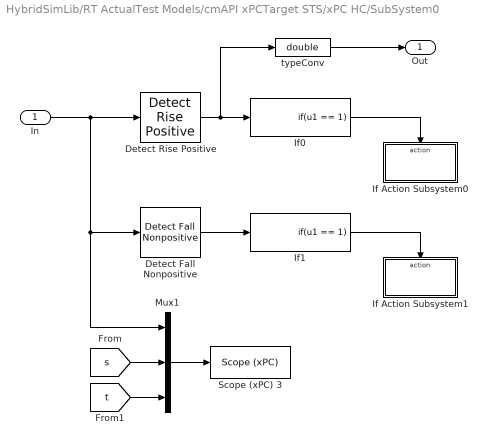
== system HybridSimLib/RT ActualTest Models/cmAPI xPCTarget STS/xPC HC/SubSystem0 ==
  In : Inport
  Detect Fall Nonpositive : simulink/Logic and Bit Operations/Detect Fall Nonpositive  vinit=0  InputProcessing=Inherited  OutDataTypeStr=uint8
  Detect Rise Positive : simulink/Logic and Bit Operations/Detect Rise Positive  vinit=0  InputProcessing=Inherited  OutDataTypeStr=uint8
  If Action Subsystem0 : Subsystem  TreatAsAtomicUnit=on
  If Action Subsystem1 : Subsystem  TreatAsAtomicUnit=on
  If0 : If  IfExpression=u1 == 1  ShowElse=off
  If1 : If  IfExpression=u1 == 1  ShowElse=off
  Mux1 : Mux  Inputs=3
  Scope (xPC) 3 : xpclib/Misc./Scope (xPC)   scopeno=7  scopetype=File  autostart=on  viewmode=Numerical  formatstr='%15.6f'  grid=on  ylimits=[0,3]  nosamples=4096  noprepostsamples=0  interleave=1  triggermode=FreeRun  triggersignal=1  triggerlevel=0.0  triggerslope=Either  triggerscope=1  triggersample=0  filename=flag.dat  mode=Lazy  writesize=512  autorestart=on  dynamicfilemode=off  maxwritefilesize=512*1024^2
  typeConv : DataTypeConversion  OutDataTypeStr=double  SaturateOnIntegerOverflow=on  RndMeth=Zero
  Out : Outport
  wires:
  [t] -> Mux1/3
  [s] -> Mux1/2
  Mux1/1 -> Scope (xPC) 3/1
  typeConv/1 -> Out/1
  If0/1 -> If Action Subsystem0/Action
  If1/1 -> If Action Subsystem1/Action
  Detect Fall Nonpositive/1 -> If1/1
  Detect Rise Positive/1 -> typeConv/1, If0/1
  In/1 -> Mux1/1, Detect Fall Nonpositive/1, Detect Rise Positive/1

== system HybridSimLib/RT ActualTest Models/cmAPI xPCTarget STS/xPC HC/SubSystem1 ==
  counter : Inport
  measDsp In : Inport  Port=2
  measFrc In : Inport  Port=3
  Hit  Crossing : HitCross  HitCrossingOffset=iDelay
  SubSystem : Subsystem  TreatAsAtomicUnit=on
  measDsp Out : Outport
  measFrc Out : Outport  Port=2
  wires:
  Hit  Crossing/1 -> SubSystem/Trigger
  counter/1 -> Hit  Crossing/1
  measDsp In/1 -> SubSystem/1(measDsp In)
  SubSystem/1(measDsp Out) -> measDsp Out/1
  measFrc In/1 -> SubSystem/2(measFrc In)
  SubSystem/2(measFrc Out) -> measFrc Out/1

== system HybridSimLib/RT ActualTest Models/cmAPI dSpace/dSpace HC/Offset/If Action ==
  In1 : Inport
  Action Port : ActionPort  PropagateVarSize=During execution
  Data Store Read : DataStoreRead  DataStoreName=x0  SampleTime=dt
  Data Store Write : DataStoreWrite  DataStoreName=x0
  Gain : Gain  Gain=1/nOffset  SaturateOnIntegerOverflow=on  OutDataTypeStr=Inherit: Same as input  ParamDataTypeStr=Inherit: Same as input
  Sum : Sum  Inputs=|++  SaturateOnIntegerOverflow=on  InputSameDT=on  OutDataTypeStr=Inherit: Same as first input
  wires:
  In1/1 -> Gain/1
  Gain/1 -> Sum/1
  Sum/1 -> Data Store Write/1
  Data Store Read/1 -> Sum/2

== system HybridSimLib/RT ActualTest Models/cmAPI dSpace/dSpace HC/Offset1/If Action ==
  In1 : Inport
  Action Port : ActionPort  PropagateVarSize=During execution
  Data Store Read : DataStoreRead  DataStoreName=x0  SampleTime=dt
  Data Store Write : DataStoreWrite  DataStoreName=x0
  Gain : Gain  Gain=1/nOffset  SaturateOnIntegerOverflow=on  OutDataTypeStr=Inherit: Same as input  ParamDataTypeStr=Inherit: Same as input
  Sum : Sum  Inputs=|++  SaturateOnIntegerOverflow=on  InputSameDT=on  OutDataTypeStr=Inherit: Same as first input
  wires:
  In1/1 -> Gain/1
  Gain/1 -> Sum/1
  Sum/1 -> Data Store Write/1
  Data Store Read/1 -> Sum/2

== system HybridSimLib/RT ActualTest Models/cmAPI dSpace/dSpace HC/SubSystem0/If Action Subsystem0 ==
  Action Port : ActionPort  PropagateVarSize=During execution
  Data Store Write0 : DataStoreWrite  DataStoreName=sFlag
  Data Store Write1 : DataStoreWrite  DataStoreName=tFlag
  atTargetFlag : Constant  Value=0  OutDataTypeStr=uint32  SampleTime=dtCon
  switchFlag : Constant  OutDataTypeStr=uint32  SampleTime=dtCon
  wires:
  switchFlag/1 -> Data Store Write0/1
  atTargetFlag/1 -> Data Store Write1/1

== system HybridSimLib/RT ActualTest Models/cmAPI dSpace/dSpace HC/SubSystem0/If Action Subsystem1 ==
  Action Port : ActionPort  PropagateVarSize=During execution
  Data Store Write0 : DataStoreWrite  DataStoreName=sFlag
  switchFlag : Constant  Value=0  OutDataTypeStr=uint32  SampleTime=dtCon
  wires:
  switchFlag/1 -> Data Store Write0/1

== system HybridSimLib/RT ActualTest Models/cmAPI dSpace/dSpace HC/SubSystem1/SubSystem ==
  measDsp In : Inport
  measFrc In : Inport  Port=2
  Trigger : TriggerPort
  Data Store Write : DataStoreWrite  DataStoreName=tFlag
  atTargetFlag : Constant  OutDataTypeStr=uint32  SampleTime=-1
  measDsp Out : Outport  InitialOutput=[0]
  measFrc Out : Outport  Port=2  InitialOutput=[0]
  wires:
  measDsp In/1 -> measDsp Out/1
  measFrc In/1 -> measFrc Out/1
  atTargetFlag/1 -> Data Store Write/1

== system HybridSimLib/RT ActualTest Models/cmAPI xPCTarget STS/xPC HC/Offset/If Action ==
  In1 : Inport
  Action Port : ActionPort  PropagateVarSize=During execution
  Data Store Read : DataStoreRead  DataStoreName=x0  SampleTime=dt
  Data Store Write : DataStoreWrite  DataStoreName=x0
  Gain : Gain  Gain=1/nOffset  SaturateOnIntegerOverflow=on  OutDataTypeStr=Inherit: Same as input  ParamDataTypeStr=Inherit: Same as input
  Sum : Sum  Inputs=|++  SaturateOnIntegerOverflow=on  InputSameDT=on  OutDataTypeStr=Inherit: Same as first input
  wires:
  In1/1 -> Gain/1
  Gain/1 -> Sum/1
  Sum/1 -> Data Store Write/1
  Data Store Read/1 -> Sum/2

== system HybridSimLib/RT ActualTest Models/cmAPI xPCTarget STS/xPC HC/Offset1/If Action ==
  In1 : Inport
  Action Port : ActionPort  PropagateVarSize=During execution
  Data Store Read : DataStoreRead  DataStoreName=x0  SampleTime=dt
  Data Store Write : DataStoreWrite  DataStoreName=x0
  Gain : Gain  Gain=1/nOffset  SaturateOnIntegerOverflow=on  OutDataTypeStr=Inherit: Same as input  ParamDataTypeStr=Inherit: Same as input
  Sum : Sum  Inputs=|++  SaturateOnIntegerOverflow=on  InputSameDT=on  OutDataTypeStr=Inherit: Same as first input
  wires:
  In1/1 -> Gain/1
  Gain/1 -> Sum/1
  Sum/1 -> Data Store Write/1
  Data Store Read/1 -> Sum/2

== system HybridSimLib/RT ActualTest Models/cmAPI xPCTarget STS/xPC HC/SubSystem0/If Action Subsystem0 ==
  Action Port : ActionPort  PropagateVarSize=During execution
  Data Store Write0 : DataStoreWrite  DataStoreName=sFlag
  Data Store Write1 : DataStoreWrite  DataStoreName=tFlag
  atTargetFlag : Constant  Value=0  SampleTime=dtCon
  switchFlag : Constant  SampleTime=dtCon
  wires:
  switchFlag/1 -> Data Store Write0/1
  atTargetFlag/1 -> Data Store Write1/1

== system HybridSimLib/RT ActualTest Models/cmAPI xPCTarget STS/xPC HC/SubSystem0/If Action Subsystem1 ==
  Action Port : ActionPort  PropagateVarSize=During execution
  Data Store Write0 : DataStoreWrite  DataStoreName=sFlag
  switchFlag : Constant  Value=0  SampleTime=dtCon
  wires:
  switchFlag/1 -> Data Store Write0/1

== system HybridSimLib/RT ActualTest Models/cmAPI xPCTarget STS/xPC HC/SubSystem1/SubSystem ==
  measDsp In : Inport
  measFrc In : Inport  Port=2
  Trigger : TriggerPort
  Data Store Write : DataStoreWrite  DataStoreName=tFlag
  atTargetFlag : Constant  SampleTime=-1
  measDsp Out : Outport  InitialOutput=[0]
  measFrc Out : Outport  Port=2  InitialOutput=[0]
  wires:
  measDsp In/1 -> measDsp Out/1
  measFrc In/1 -> measFrc Out/1
  atTargetFlag/1 -> Data Store Write/1

== stateflow chart RT ActualTest Models/cmAPI dSpace/dSpace HC/Predictor-Corrector ==
  state HybridController [parallel]
    settings: executionOrder=1
    state Predict
      en: state = 1;
      en: diSD = 1;
      en: i = 1; iSD = 0;
      en: predictD3(&com,i/N);
      du: i++;
      du: predictD3(&com,i/N);
    state Initialize
      en: i = 1; iSD = 0;
      en: diSD = 1;
      en: initData(nAct,dtCon);
      en: zeroDsp(&com);
    state AutoSlowDown
      en: state = 2;
      en: diSD = 4-i/(0.2*N);
      en: i += diSD; iSD = i;
      en: predictD3(&com,i/N);
      du: diSD = 4-i/(0.2*N);
      du: i += diSD; iSD = i;
      du: predictD3(&com,i/N);
    state Correct
      en: state = 0;
      en: setCurDsp(&com,i/N);
      en: dspLocal = dsp; setNewDsp(&dspLocal);
      en: di = min(max(diSD+1/(0.2*N)*(i-iSD),0.001),1.0);
      en: i = min(i+di,N);
      en: correctD3(&com,i/N);
      du: di = min(max(diSD+1/(0.2*N)*(i-iSD),0.001),1.0);
      du: i = min(i+di,N);
      du: correctD3(&com,i/N);
    Correct -> Predict : [i>=N]
    (default) -> Initialize
    Predict -> Correct [order 2] : [flag==1]
    Initialize -> Correct : [flag==1]
    AutoSlowDown -> Correct : [flag==1]
    Predict -> AutoSlowDown [order 1] : [i>=0.6*N && flag~=1]
  data: dsp input double size=nAct; flag input uint32; com output double size=nAct; state output uint32; i output double; N local double; nAct parameter uint32 =1; iDelay local double; di local double; diSD local double; iSD local double; dspLocal local double size=nAct

== stateflow chart RT ActualTest Models/cmAPI xPCTarget STS/xPC HC/Predictor-Corrector ==
  state HybridController [parallel]
    settings: executionOrder=1
    state Predict
      en: state = 1;
      en: setCurDsp(&com,i/N);
      en: diSD = 1;
      en: i = 1; iSD = 0;
      en: predictD3(&com,i/N);
      du: i++;
      du: predictD3(&com,i/N);
    state Initialize
      en: i = 1; iSD = 0;
      en: diSD = 1;
      en: initData(nAct,dtCon);
      en: zeroDsp(&com);
    state AutoSlowDown
      en: state = 2;
      en: diSD = 4-i/(0.2*N);
      en: i += diSD; iSD = i;
      en: predictD3(&com,i/N);
      du: diSD = 4-i/(0.2*N);
      du: i += diSD; iSD = i;
      du: predictD3(&com,i/N);
    state Correct
      en: state = 0;
      en: setCurDsp(&com,i/N);
      en: dspLocal = dsp; setNewDsp(&dspLocal);
      en: di = min(max(diSD+1/(0.2*N)*(i-iSD),0.001),1.0);
      en: i = min(i+di,N);
      en: correctD3(&com,i/N);
      du: di = min(max(diSD+1/(0.2*N)*(i-iSD),0.001),1.0);
      du: i = min(i+di,N);
      du: correctD3(&com,i/N);
    Correct -> Predict : [i>=N]
    (default) -> Initialize
    Predict -> Correct [order 2] : [flag==1]
    Initialize -> Correct : [flag==1]
    AutoSlowDown -> Correct : [flag==1]
    Predict -> AutoSlowDown [order 1] : [i>=0.6*N && flag~=1]
  data: dsp input double size=nAct; flag input double size=1; com output double size=nAct; state output double size=1; i output double size=1; N local double size=1; nAct parameter double size=1 =1; iDelay local double size=1; di local double size=1; diSD local double size=1; iSD local double size=1; dspLocal local double size=nAct
